simulink library "BatteryLibrary_lib_YL"  (R2023b)
settings: Solver=VariableStepAuto  StartTime=0.0  StopTime=10.0  RelTol=1e-3
undefined symbols (not defined in the file): stopState
settings Model: Creator=yili  LastModifiedBy=Yi.Li

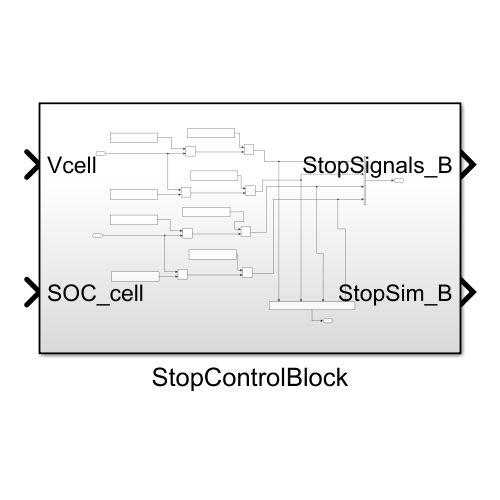
[thumbnail: Simulink's stored preview of the top-level diagram]
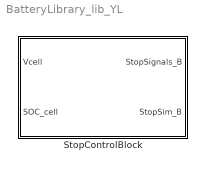
== system BatteryLibrary_lib_YL ==
  StopControlBlock : Subsystem

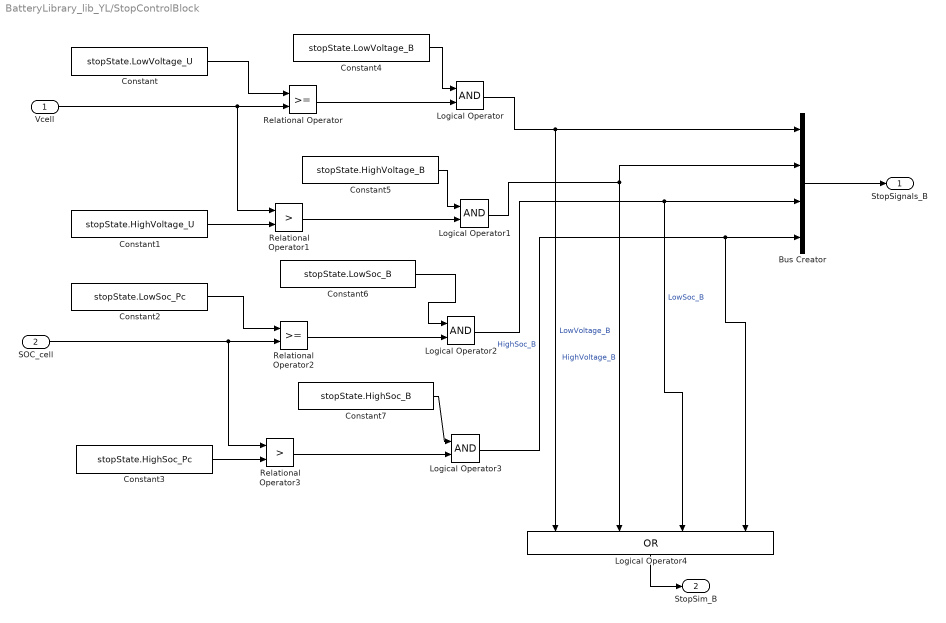
== system BatteryLibrary_lib_YL/StopControlBlock ==
  Vcell : Inport
  SOC_cell : Inport  Port=2
  Bus Creator : BusCreator  Inputs=4
  Constant : Constant  Value=stopState.LowVoltage_U
  Constant1 : Constant  Value=stopState.HighVoltage_U
  Constant2 : Constant  Value=stopState.LowSoc_Pc
  Constant3 : Constant  Value=stopState.HighSoc_Pc
  Constant4 : Constant  Value=stopState.LowVoltage_B
  Constant5 : Constant  Value=stopState.HighVoltage_B
  Constant6 : Constant  Value=stopState.LowSoc_B
  Constant7 : Constant  Value=stopState.HighSoc_B
  Logical Operator{,1..3} (4 alike) : Logic  AllPortsSameDT=off  OutDataTypeStr=boolean
  Logical Operator4 : Logic  Operator=OR  Inputs=4  AllPortsSameDT=off  OutDataTypeStr=boolean
  Relational Operator : RelationalOperator  OutDataTypeStr=boolean  RndMeth=Simplest  InputSameDT=off
  Relational Operator1 : RelationalOperator  Operator=>  OutDataTypeStr=boolean  RndMeth=Simplest  InputSameDT=off
  Relational Operator2 : RelationalOperator  OutDataTypeStr=boolean  RndMeth=Simplest  InputSameDT=off
  Relational Operator3 : RelationalOperator  Operator=>  OutDataTypeStr=boolean  RndMeth=Simplest  InputSameDT=off
  StopSignals_B : Outport
  StopSim_B : Outport  Port=2
  wires:
  Vcell/1 -> Relational Operator/2, Relational Operator1/1
  Logical Operator/1 -> Bus Creator/1, Logical Operator4/1  "LowVoltage_B"
  Logical Operator2/1 -> Bus Creator/3, Logical Operator4/3  "LowSoc_B"
  Constant/1 -> Relational Operator/1
  Logical Operator3/1 -> Logical Operator4/4, Bus Creator/4  "HighSoc_B"
  Logical Operator4/1 -> StopSim_B/1
  Logical Operator1/1 -> Bus Creator/2, Logical Operator4/2  "HighVoltage_B"
  Constant7/1 -> Logical Operator3/1
  Constant3/1 -> Relational Operator3/2
  SOC_cell/1 -> Relational Operator2/2, Relational Operator3/1
  Constant2/1 -> Relational Operator2/1
  Relational Operator2/1 -> Logical Operator2/2
  Relational Operator3/1 -> Logical Operator3/2
  Constant6/1 -> Logical Operator2/1
  Constant4/1 -> Logical Operator/1
  Relational Operator1/1 -> Logical Operator1/2
  Relational Operator/1 -> Logical Operator/2
  Constant1/1 -> Relational Operator1/2
  Constant5/1 -> Logical Operator1/1
  Bus Creator/1 -> StopSignals_B/1
